simulink model "Controllori"  (R2020b)
settings: Solver=VariableStepAuto  StartTime=0.0  StopTime=10.0  RelTol=1e-3
values from neighbouring files (symbols this model uses):
  A_num = eval(A)    [eq_non_linear.m]
  B_num = eval(B)    [eq_non_linear.m]
  C_num = eval(C)    [eq_non_linear.m]
  D_num = eval(D)    [eq_non_linear.m]
  G0_fb_R = dcgain(reg_fb_R)    [controllo.m]
  G0_fb_Y = dcgain(reg_fb_Y)    [controllo.m]
  G0_fb_z = dcgain(reg_fb_z)    [controllo.m]
  reg_dir_R = ss(A_R-B_R*K_R-L_R*C_R,L_R,K_R,0)    [controllo.m]
  reg_dir_Y = ss(A_Y-B_Y*K_Y-L_Y*C_Y,L_Y,K_Y,0)    [controllo.m]
  reg_dir_z = ss(A_z-B_z*K_z-L_z*C_z,L_z,K_z,0)    [controllo.m]
  reg_fb_R = ss(A_R-B_R*K_R-L_R*C_R,-L_R,-K_R,0)    [controllo.m]
  reg_fb_Y = ss(A_Y-B_Y*K_Y-L_Y*C_Y,-L_Y,-K_Y,0)    [controllo.m]
  reg_fb_z = ss(A_z-B_z*K_z-L_z*C_z,-L_z,-K_z,0)    [controllo.m]
libraries: simulink x1
settings Model: Creator=Tommaso  LastModifiedBy=Tommaso

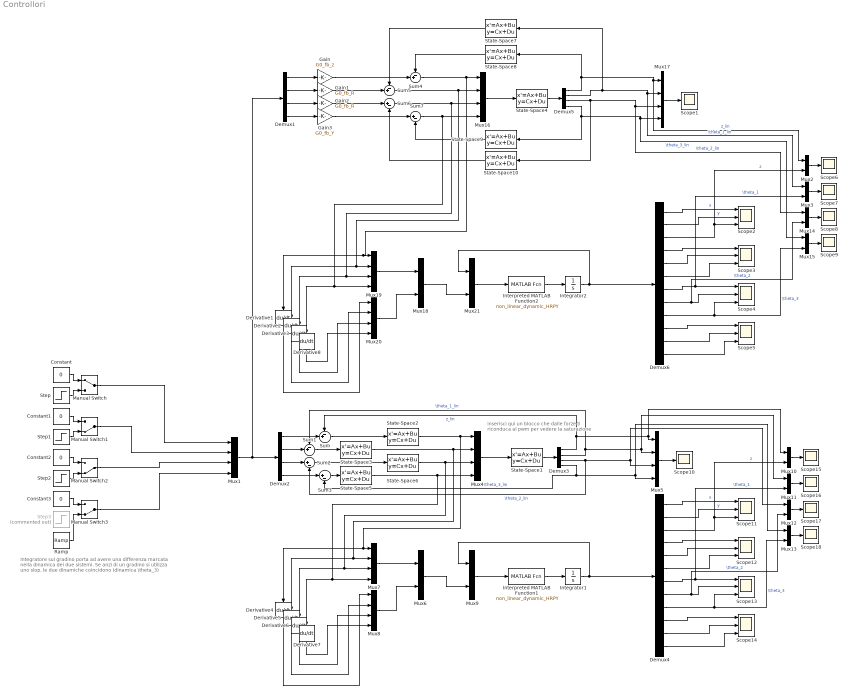
== system Controllori ==
  note: inserisci qui un blocco che dalle forze ti
      | riconduca al pwm per vedere la saturazione
  note: Integratore sul gradino porta ad avere una differenza
      | marcata nella dinamica dei due sistemi. Se anzi di un gradino
      | si utilizza uno slop, le due dinamiche coincidono
      | (dinamica \theta_3)
  Constant{,1..3} (4 alike) : Constant  Value=0
  Demux{1..3,5} (4 alike) : Demux
  Demux4 : Demux  Outputs=12
  Demux6 : Demux  Outputs=12
  Derivative{1..8} (8 alike) : Derivative
  Gain : Gain  Gain=G0_fb_z
  Gain1 : Gain  Gain=G0_fb_R
  Gain2 : Gain  Gain=G0_fb_R
  Gain3 : Gain  Gain=G0_fb_Y
  Integrator1 : Integrator  InitialCondition=[0,0,0,0,0,0,0,0,0,0,0,0]
  Integrator2 : Integrator  InitialCondition=[0,0,0,0,0,0,0,0,0,0,0,0]
  Interpreted MATLAB Function1 : MATLABFcn  MATLABFcn=non_linear_dynamic_HRPY
  Interpreted MATLAB Function2 : MATLABFcn  MATLABFcn=non_linear_dynamic_HRPY
  Manual Switch : ManualSwitch
  Manual Switch1 : ManualSwitch  CurrentSetting=0
  Manual Switch2 : ManualSwitch  CurrentSetting=0
  Manual Switch3 : ManualSwitch  CurrentSetting=0
  Mux{1,4..5,7..8,16..17,19..20} (9 alike) : Mux
  Mux{2..3,6,9..15,18,21} (12 alike) : Mux  Inputs=2
  Ramp : simulink/Sources/Ramp  slope=0.1  start=1  InitialOutput=0
  Scope{1,6..10,15..18} (10 alike) : Scope
  Scope{2..5,11..14} (8 alike) : Scope  NumInputPorts=3
  State-Space1 : StateSpace  A=A_num  B=B_num  C=C_num  D=D_num  InitialCondition=0
  State-Space10 : StateSpace  A=reg_fb_R.a  B=reg_fb_R.b  C=reg_fb_R.c  D=reg_fb_R.d  InitialCondition=0
  State-Space2 : StateSpace  A=reg_dir_z.a  B=reg_dir_z.b  C=reg_dir_z.c  D=reg_dir_z.d  InitialCondition=0
  State-Space3 : StateSpace  A=reg_dir_R.a  B=reg_dir_R.b  C=reg_dir_R.c  D=reg_dir_R.d  InitialCondition=0
  State-Space4 : StateSpace  A=A_num  B=B_num  C=C_num  D=D_num  InitialCondition=0
  State-Space5 : StateSpace  A=reg_dir_Y.a  B=reg_dir_Y.b  C=reg_dir_Y.c  D=reg_dir_Y.d  InitialCondition=0
  State-Space6 : StateSpace  A=reg_dir_R.a  B=reg_dir_R.b  C=reg_dir_R.c  D=reg_dir_R.d  InitialCondition=0
  State-Space7 : StateSpace  A=reg_fb_R.a  B=reg_fb_R.b  C=reg_fb_R.c  D=reg_fb_R.d  InitialCondition=0
  State-Space8 : StateSpace  A=reg_fb_z.a  B=reg_fb_z.b  C=reg_fb_z.c  D=reg_fb_z.d  InitialCondition=0
  State-Space9 : StateSpace  A=reg_fb_Y.a  B=reg_fb_Y.b  C=reg_fb_Y.c  D=reg_fb_Y.d  InitialCondition=0
  Step : Step  After=3  SampleTime=0
  Step1 : Step  After=0.1  SampleTime=0
  Step2 : Step  After=0.1  SampleTime=0
  Step3 : Step  Commented=on  After=0.1  SampleTime=0
  Sum{,1,4..5} (4 alike) : Sum  Inputs=-+|
  Sum{2..3,6..7} (4 alike) : Sum  Inputs=|+-
  wires:
  Demux4/4 -> Scope12/1
  Demux4/11 -> Scope14/2
  State-Space2/1 -> Derivative4/1, Mux7/1, Mux4/1
  Demux4/8 -> Mux12/2, Scope13/2  "\\theta_2"
  Demux2/3 -> Sum2/1
  Mux7/1 -> Mux6/1
  Mux11/1 -> Scope16/1
  Demux4/12 -> Scope14/3
  Demux4/7 -> Mux11/2, Scope13/1  "\\theta_1"
  Mux13/1 -> Scope18/1
  Integrator1/1 -> Mux9/1, Demux4/1
  Mux12/1 -> Scope17/1
  Mux10/1 -> Scope15/1
  State-Space1/1 -> Demux3/1
  Sum/1 -> State-Space2/1
  Interpreted MATLAB Function1/1 -> Integrator1/1
  Demux4/10 -> Scope14/1
  Demux4/5 -> Scope12/2
  Demux4/6 -> Scope12/3
  Demux4/3 -> Mux10/2, Scope11/3  "z"
  Mux9/1 -> Interpreted MATLAB Function1/1
  Mux8/1 -> Mux6/2
  Manual Switch3/1 -> Mux1/4
  Demux4/9 -> Mux13/2, Scope13/3  "\\theta_3"
  Mux4/1 -> State-Space1/1
  Derivative4/1 -> Mux8/1
  Sum2/1 -> State-Space6/1
  Derivative5/1 -> Mux8/2
  Constant2/1 -> Manual Switch2/1
  Mux5/1 -> Scope10/1
  Demux4/2 -> Scope11/2  "y"
  Demux3/1 -> Sum/1, Mux10/1, Mux5/1  "z_lin"
  Mux6/1 -> Mux9/2
  Sum1/1 -> State-Space3/1
  Sum3/1 -> State-Space5/1
  State-Space5/1 -> Mux7/4, Derivative7/1, Mux4/4
  Derivative6/1 -> Mux8/3
  Demux2/4 -> Sum3/1
  State-Space6/1 -> Mux7/3, Derivative6/1, Mux4/3
  Demux4/1 -> Scope11/1  "x"
  State-Space3/1 -> Derivative5/1, Mux7/2, Mux4/2
  Demux3/3 -> Sum2/2, Mux5/3, Mux12/1  "\\theta_2_lin"
  Demux3/4 -> Mux13/1, Mux5/4, Sum3/2  "\\theta_3_lin"
  Demux2/2 -> Sum1/2
  Derivative7/1 -> Mux8/4
  Demux3/2 -> Mux11/1, Mux5/2, Sum1/1  "\\theta_1_lin"
  Demux2/1 -> Sum/2
  Step2/1 -> Manual Switch2/2
  Constant/1 -> Manual Switch/1
  Manual Switch1/1 -> Mux1/2
  Manual Switch2/1 -> Mux1/3
  Constant1/1 -> Manual Switch1/1
  Step1/1 -> Manual Switch1/2
  Constant3/1 -> Manual Switch3/1
  Ramp/1 -> Manual Switch3/2
  Manual Switch/1 -> Mux1/1
  Step/1 -> Manual Switch/2
  Sum4/1 -> Derivative1/1, Mux19/1, Mux16/1
  Derivative8/1 -> Mux20/4
  Demux5/2 -> Mux3/1, Mux17/2, State-Space7/1  "\\theta_1_lin"
  Demux5/3 -> State-Space10/1, Mux17/3, Mux14/1  "\\theta_2_lin"
  Demux5/4 -> Mux15/1, Mux17/4, State-Space9/1  "\\theta_3_lin"
  Sum5/1 -> Derivative2/1, Mux19/2, Mux16/2
  Sum6/1 -> Derivative3/1, Mux19/3, Mux16/3
  Derivative3/1 -> Mux20/3
  Demux6/2 -> Scope2/2  "y"
  Demux5/1 -> State-Space8/1, Mux2/1, Mux17/1  "z_lin"
  Mux21/1 -> Interpreted MATLAB Function2/1
  Demux6/6 -> Scope3/3
  Mux17/1 -> Scope1/1
  Demux6/3 -> Mux2/2, Scope2/3  "z"
  Mux20/1 -> Mux18/2
  Interpreted MATLAB Function2/1 -> Integrator2/1
  Integrator2/1 -> Mux21/1, Demux6/1
  Mux16/1 -> State-Space4/1
  State-Space4/1 -> Demux5/1
  Demux6/5 -> Scope3/2
  Mux14/1 -> Scope8/1
  Mux2/1 -> Scope6/1
  Demux6/10 -> Scope5/1
  Demux6/1 -> Scope2/1  "x"
  Mux15/1 -> Scope9/1
  Demux6/9 -> Mux15/2, Scope4/3  "\\theta_3"
  Derivative2/1 -> Mux20/2
  Demux6/12 -> Scope5/3
  Mux19/1 -> Mux18/1
  Mux18/1 -> Mux21/2
  Derivative1/1 -> Mux20/1
  Sum7/1 -> Derivative8/1, Mux19/4, Mux16/4
  Demux6/8 -> Mux14/2, Scope4/2  "\\theta_2"
  Mux3/1 -> Scope7/1
  Mux1/1 -> Demux1/1, Demux2/1
  Demux6/4 -> Scope3/1
  Demux6/11 -> Scope5/2
  Demux6/7 -> Mux3/2, Scope4/1  "\\theta_1"
  State-Space7/1 -> Sum5/1
  State-Space8/1 -> Sum4/1
  State-Space9/1 -> Sum7/2
  State-Space10/1 -> Sum6/2
  Demux1/4 -> Gain3/1
  Demux1/3 -> Gain2/1
  Demux1/2 -> Gain1/1
  Demux1/1 -> Gain/1
  Gain/1 -> Sum4/2
  Gain1/1 -> Sum5/2
  Gain2/1 -> Sum6/1
  Gain3/1 -> Sum7/1
